simulink model "test_InvDyn"  (Simulink 7.9)
settings: Solver=FixedStepDiscrete  StartTime=0.0  StopTime=inf  FixedStep=1  RelTol=1e-3
libraries: WBCLibrary x2
settings Model: Creator=jorhabib  LastModifiedBy=jorhabib

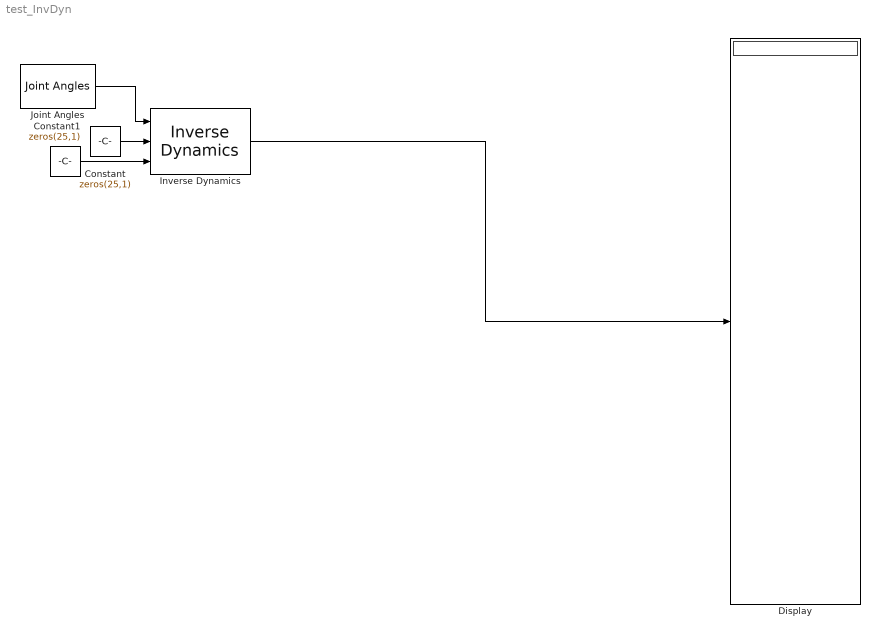
== system test_InvDyn ==
  Constant : Constant  Value=zeros(25,1)  OutDataTypeStr=double  SampleTime=-1
  Constant1 : Constant  Value=zeros(25,1)  OutDataTypeStr=double  SampleTime=-1
  Display : Display
  Inverse Dynamics : WBCLibrary/wholeBodyModel/Dynamics/Inverse Dynamics  robotName=robotName  localName=localName
  Joint Angles : WBCLibrary/wholeBodyStates/Joint Angles  robotName=robotName  localName=localName
  wires:
  Joint Angles/1 -> Inverse Dynamics/1
  Constant/1 -> Inverse Dynamics/2
  Constant1/1 -> Inverse Dynamics/3
  Inverse Dynamics/1 -> Display/1
